simulink model "NREL_Diesel_Genset_Test_System"  (Simulink 8.1)
settings: Solver=ode3  SolverMode=SingleTasking  StartTime=0.0  StopTime=Stim.Trep  FixedStep=Ts  RelTol=1e-3
PostLoadFcn:
  | Ts=100e-6;GenSelect='3.5MW';initGTS;
InitFcn:
  | Ts=100e-6;GenSelect='3.5MW';initGTS;
values from neighbouring files (symbols this model uses):
  GenMult = 1    [initGTS.m]
  GenPN = 3.5e6    (= 3500000)    [initGTS.m]
  GenVN = 13800    [initGTS.m]
undefined symbols (not defined in the file or in its folder): breakers_1ph_3ph, CBID, DER_REL, DiscIntNeverNeededParam, Efd0, Efd1, Efd2, F3, Gen_900kW_external_control, HIL_GenSet, Ka, Ke, Kf, Protection, SeEfd1, SeEfd2, Stim, Ta, Te, Tf, VR0, VRmax, VRmin
libraries: powerlib x33, powerlib_extras x10, simulink x9, PQFV_lib x2, rtlab x2, cables_lib x2, breaker_lib x2, NREL_Diesel_Genset_lib x2, relay_modbus_lib x2, powerlib_models x1
(part 2 of 2)

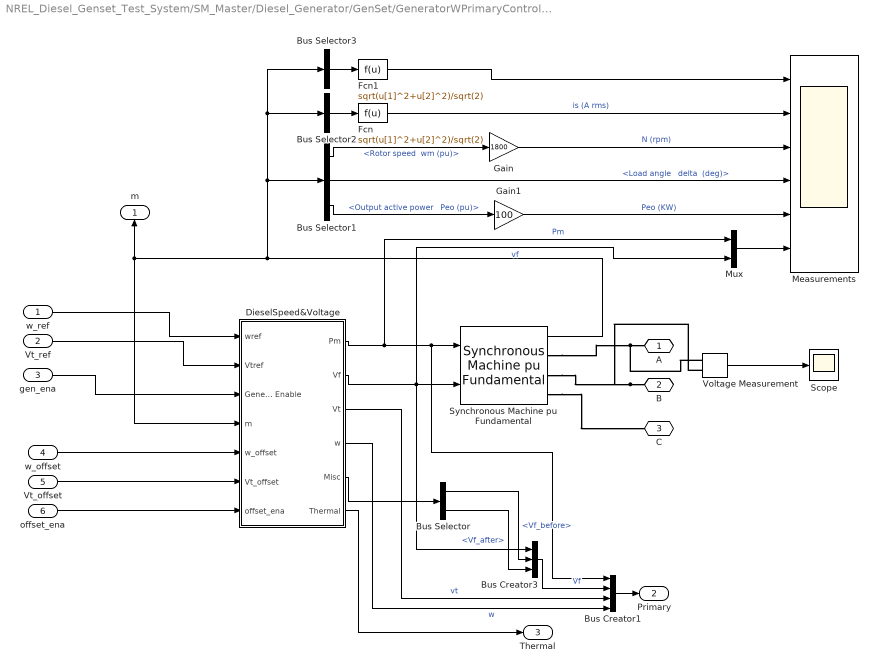
== system NREL_Diesel_Genset_Test_System/SM_Master/Diesel_Generator/GenSet/GeneratorWPrimaryControllers ==
  w_ref : Inport
  Vt_ref : Inport  Port=2
  gen_ena : Inport  Port=3
  w_offset : Inport  Port=4
  Vt_offset : Inport  Port=5
  offset_ena : Inport  Port=6
  Bus Creator1 : BusCreator
  Bus Creator3 : BusCreator  Inputs=3
  Bus Selector : BusSelector  OutputSignals=Vf_before,Vf_after
  Bus Selector1 : BusSelector  OutputSignals="Mechanical.Rotor speed  wm (pu),Load angle   delta  (deg),Output active power   Peo (pu)"
  Bus Selector2 : BusSelector  OutputSignals="dq0 components.Stator current  iq (pu),dq0 components.Stator current  id (pu)"  OutputAsBus=on
  Bus Selector3 : BusSelector  OutputSignals="dq0 components.Stator voltage  vq (pu),dq0 components.Stator voltage  vd (pu)"  OutputAsBus=on
  DieselSpeed&Voltage : Subsystem
  Fcn : Fcn  Expr=sqrt(u[1]^2+u[2]^2)/sqrt(2)
  Fcn1 : Fcn  Expr=sqrt(u[1]^2+u[2]^2)/sqrt(2)
  Gain : Gain  Gain=1800  SaturateOnIntegerOverflow=on  OutDataTypeStr=Inherit: Same as input  ParamDataTypeStr=Inherit: Same as input
  Gain1 : Gain  Gain=100  SaturateOnIntegerOverflow=on  OutDataTypeStr=Inherit: Same as input  ParamDataTypeStr=Inherit: Same as input
  Measurements : Scope  NumInputPorts=6
      settings: TickLabels=on  TimeRange=3  YMin=0~0~0~-200~-2.5e+18~-0.05  YMax=7e+08~1e+08~2.75e+08~200~1.25e+19~0.2  SaveName=is
  Mux : Mux  Inputs=2
  Scope : Scope
      settings: YMin=-750  YMax=750  SaveName=ScopeData12  Decimation=10
  Synchronous Machine pu Fundamental : powerlib/Machines/Synchronous Machine pu Fundamental  PresetModel=No  MechanicalLoad=Mechanical power Pm  ShowDetailedParameters=on  RotorType=Salient-pole  NominalParameters=[GP.Pn GP.Vn GP.fn]  Stator=GP.Stator  Field=GP.Field  Dampers2=[0.0652, 0.5134, 0.0287, 0.2553, 7.765e-3, 0.9167 ]  Dampers1=GP.Dampers  Mechanical=GP.Inertia  PolePairs=2  InitialConditions=GP.Initial  SetSaturation=off  Saturation=[0.6404,0.7127,0.8441,0.9214,0.9956,1.082,1.19,1.316,1.457;0.7,0.7698,0.8872,0.9466,0.9969,1.046,1.1,1.151,1.201]  Units=per unit fundamental parameters  LoadFlowParameters=[1,0,0,0,0]  TsPowergui=0  TsBlock=-1  IterativeModel=Trapezoidal non iterative  BusType=swing  Pref=0  Qref=0  Qmin=-inf  Qmax=inf  PLF=0  QLF=0
  Voltage Measurement : powerlib/Measurements/Voltage Measurement  PhasorSimulation=off  OutputType=Complex  PSBequivalent=0
  A : PMIOPort  Port=1  Side=Right
  B : PMIOPort  Port=2  Side=Right
  C : PMIOPort  Port=3  Side=Right
  m : Outport
  Primary : Outport  Port=2
  Thermal : Outport  Port=3
  wires:
  offset_ena/1 -> DieselSpeed&Voltage/7(offset_ena)
  Vt_offset/1 -> DieselSpeed&Voltage/6(Vt_offset)
  w_offset/1 -> DieselSpeed&Voltage/5(w_offset)
  Voltage Measurement/1 -> Scope/1
  Mux/1 -> Measurements/6
  Fcn1/1 -> Measurements/1
  Bus Selector3/1 -> Fcn1/1
  Bus Selector1/1 -> Gain/1  "<Rotor speed  wm (pu)>"
  Bus Selector1/2 -> Measurements/4  "<Load angle   delta  (deg)>"
  Bus Selector1/3 -> Gain1/1  "<Output active power   Peo (pu)>"
  Gain1/1 -> Measurements/5  "Peo (KW)"
  Gain/1 -> Measurements/3  "N (rpm)"
  Bus Selector2/1 -> Fcn/1
  Fcn/1 -> Measurements/2  "is (A rms)"
  Vt_ref/1 -> DieselSpeed&Voltage/2(Vtref)
  w_ref/1 -> DieselSpeed&Voltage/1(wref)
  DieselSpeed&Voltage/2(Vf) -> Synchronous Machine pu Fundamental/2, Mux/2, Bus Creator3/1  "vf"
  DieselSpeed&Voltage/1(Pm) -> Bus Creator1/1, Synchronous Machine pu Fundamental/1, Mux/1  "Pm"
  gen_ena/1 -> DieselSpeed&Voltage/3(Generator Enable)
  Synchronous Machine pu Fundamental/1 -> m/1, DieselSpeed&Voltage/4(m), Bus Selector3/1, Bus Selector2/1, Bus Selector1/1
  DieselSpeed&Voltage/3(Vt) -> Bus Creator1/3  "vt"
  DieselSpeed&Voltage/4(w) -> Bus Creator1/4  "w"
  Bus Creator1/1 -> Primary/1
  DieselSpeed&Voltage/5(Misc) -> Bus Selector/1
  Bus Selector/1 -> Bus Creator3/2  "<Vf_before>"
  Bus Selector/2 -> Bus Creator3/3  "<Vf_after>"
  Bus Creator3/1 -> Bus Creator1/2  "Vf"
  DieselSpeed&Voltage/6(Thermal) -> Thermal/1
  connections:
  Synchronous Machine pu Fundamental/RConn3 -- C/RConn1
  B/RConn1 -- Voltage Measurement/LConn2 -- Synchronous Machine pu Fundamental/RConn2
  A/RConn1 -- Voltage Measurement/LConn1 -- Synchronous Machine pu Fundamental/RConn1

== system NREL_Diesel_Genset_Test_System/SM_Master/Diesel_Generator/GenSet/NumOscillation ==
  Ground2 : powerlib/Elements/Ground  LConnTagsString=a
  "RLC " : powerlib/Elements/Parallel RLC Branch  LConnTagsString=a  RConnTagsString=__new0  BranchType=R  Resistance=10e6  Inductance=inf  SetiL0=off  InitialCurrent=0  Capacitance=10e-6  Setx0=off  InitialVoltage=0  Measurements=None
  RLC1 : powerlib/Elements/Parallel RLC Branch  LConnTagsString=a  RConnTagsString=__new0  BranchType=R  Resistance=10e6  Inductance=inf  SetiL0=off  InitialCurrent=0  Capacitance=10e-6  Setx0=off  InitialVoltage=0  Measurements=None
  RLC2 : powerlib/Elements/Parallel RLC Branch  LConnTagsString=a  RConnTagsString=__new0  BranchType=R  Resistance=10e6  Inductance=inf  SetiL0=off  InitialCurrent=0  Capacitance=10e-6  Setx0=off  InitialVoltage=0  Measurements=None
  RLC3 : powerlib/Elements/Parallel RLC Branch  LConnTagsString=a  RConnTagsString=__new0  BranchType=R  Resistance=10e-3  Inductance=inf  SetiL0=off  InitialCurrent=0  Capacitance=0  Setx0=off  InitialVoltage=0  Measurements=None
  RLC4 : powerlib/Elements/Parallel RLC Branch  LConnTagsString=a  RConnTagsString=__new0  BranchType=R  Resistance=10e-3  Inductance=inf  SetiL0=off  InitialCurrent=0  Capacitance=0  Setx0=off  InitialVoltage=0  Measurements=None
  RLC5 : powerlib/Elements/Parallel RLC Branch  LConnTagsString=a  RConnTagsString=__new0  BranchType=R  Resistance=10e-3  Inductance=inf  SetiL0=off  InitialCurrent=0  Capacitance=0  Setx0=off  InitialVoltage=0  Measurements=None
  A : PMIOPort  Port=1  Side=Left
  B : PMIOPort  Port=2  Side=Left
  C : PMIOPort  Port=3  Side=Left
  connections:
  C/RConn1 -- RLC5/LConn1
  B/RConn1 -- RLC4/LConn1
  A/RConn1 -- RLC3/LConn1
  RLC3/RConn1 -- RLC2/LConn1
  RLC1/LConn1 -- RLC4/RConn1
  "RLC "/LConn1 -- RLC5/RConn1
  RLC2/RConn1 -- Ground2/LConn1 -- RLC1/RConn1 -- "RLC "/RConn1

== system NREL_Diesel_Genset_Test_System/SM_Master/Diesel_Generator/GenSet/StabilityL ==
  Constant Load : powerlib/Elements/Three-Phase Parallel RLC Load  LConnTagsString=A|B|C  Configuration=Y (grounded)  NominalVoltage=v  NominalFrequency=60  ActivePower=kVA*1E3*pf  InductivePower=kVA*1E3*sqrt(1-pf^2)  CapacitivePower=0  Measurements=None  LoadType=constant Z
  A : PMIOPort  Port=1  Side=Left
  B : PMIOPort  Port=2  Side=Left
  C : PMIOPort  Port=3  Side=Left
  connections:
  A/RConn1 -- Constant Load/LConn1
  B/RConn1 -- Constant Load/LConn2
  C/RConn1 -- Constant Load/LConn3

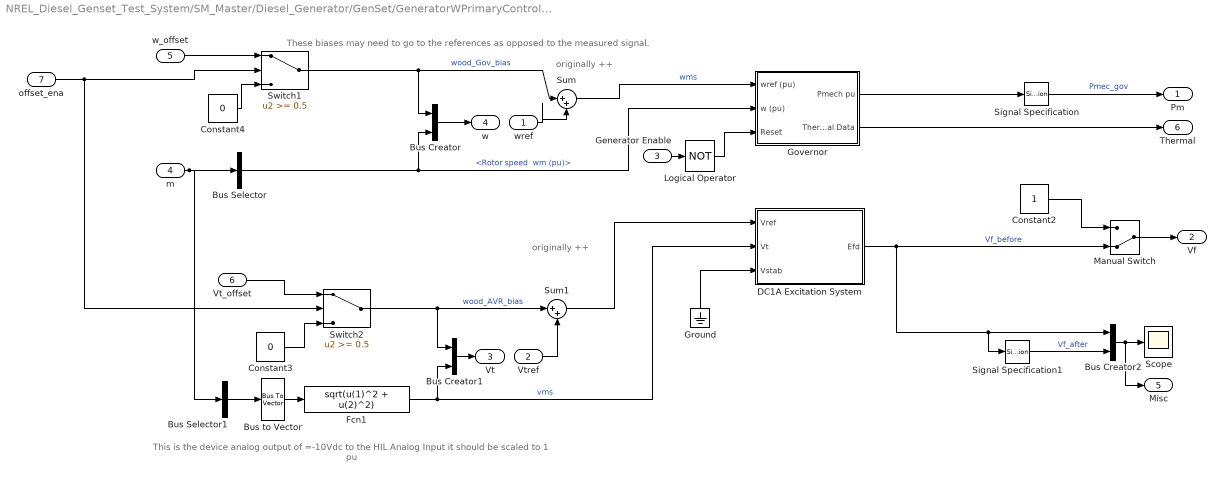
== system NREL_Diesel_Genset_Test_System/SM_Master/Diesel_Generator/GenSet/GeneratorWPrimaryControllers/DieselSpeed&Voltage ==
  note: This is the device analog output of =-10Vdc to
      | the HIL Analog Input it should be scaled to 1 pu
  note: These biases may need to
      | go to the references as opposed
      | to the measured signal.
  note: originally ++
  note: originally ++
  wref : Inport  SampleTime=Ts
  Vtref : Inport  Port=2  SampleTime=Ts
  Generator Enable : Inport  Port=3  SampleTime=Ts
  m : Inport  Port=4  SampleTime=Ts
  w_offset : Inport  Port=5
  Vt_offset : Inport  Port=6
  offset_ena : Inport  Port=7
  Bus Creator : BusCreator  Inputs=2
  Bus Creator1 : BusCreator  Inputs=2
  Bus Creator2 : BusCreator  Inputs=2
  Bus Selector : BusSelector  OutputSignals="Mechanical.Rotor speed  wm (pu)"
  Bus Selector1 : BusSelector  OutputSignals="dq0 components.Stator voltage  vd (pu),dq0 components.Stator voltage  vq (pu)"  OutputAsBus=on
  Bus to Vector : BusToVector
  Constant2 : Constant
  Constant3 : Constant  Value=0
  Constant4 : Constant  Value=0
  DC1A Excitation System : Subsystem  AncestorBlock=sps_avr/DC1A Excitation System  mask(DC1A Excitation System){Tr=GP.Ex.Tr, KaTa=GP.Ex.Regulator, VRminmax=[0 8], KfTf=GP.Ex.Damping, TbTc=[0 0], KeTe=GP.Ex.Exciter, Efd12=[6.83 6.08], SeEfd12=[ 0.132 0.062], v0=[0 0], TsBlock=Ts}
      mask prompts: Tr "Low-pass filter time constant Tr(s):"; KaTa "Voltage regulator gain and time constant [Ka Ta(s)]:"; VRminmax "Voltage regulator output limits [VRmin(pu) VRmax(pu)]:"; KfTf "Damping filter gain and time constant [Kf Tf(s)]:"; TbTc "Transient gain reduction lead and lag time constants [Tb(s) Tc(s)]:"; KeTe "Exciter gain and time constant [Ke Te(s)]:"; Efd12 "Field voltage values [Efd1(pu) Efd2(pu)]:"; SeEfd12 "Exciter saturation function values [SeEfd1(pu) SeEfd2(pu)]:"; v0 "Initial values of terminal voltage and field voltage [Vt0(pu) Efd0(pu)]:"; TsBlock "Sample time:"
      mask help: Implements a synchronous machine voltage regulator and exciter based on the IEEE type DC1A excitation system model. The output is the field voltage to apply to the Vf input of a Synchronous Machine block. Inputs and output are in p.u.
      mask init:
      | block = gcb;
      | [Ts,BlockChoice,MaskType,Ka,Ta,Ke,Te,Kf,Tf,Tb,Tc,Efd1,Efd2,SeEfd1,SeEfd2,VRmin,VRmax,Vt0,Efd0,VR0] = powericon('ExcitationSystemInit',block,TsBlock,KaTa,KeTe,KfTf,TbTc,Efd12,SeEfd12,VRminmax,v0);
      | %powericon('SetInternalModels','set',block,BlockChoice);
      mask Help: helpview(psbhelp);
      mask Display: color('blue');disp('DC1A')
  Fcn1 : Fcn  Expr=sqrt(u(1)^2 + u(2)^2)
  Governor : Subsystem  BlockChoice=GEJenbacherJ620
      settings: AttributesFormatString=%<BlockChoice>  MemberBlocks=DieselGovernor,GEJenbacherJ620
      settings: TemplateBlock=|
      | NREL_Diesel_Genset_lib/Configurable
      | Subsystem
  Ground : Ground
  Logical Operator : Logic  Operator=NOT  AllPortsSameDT=off  OutDataTypeStr=boolean
  Manual Switch : ManualSwitch  CurrentSetting=0
  Scope : Scope
      settings: YMin=1.0475  YMax=1.08
  Signal Specification : SignalSpecification  Dimensions=1
  Signal Specification1 : SignalSpecification  Dimensions=1
  Sum : Sum  Inputs=|++
  Sum1 : Sum  Inputs=|++
  Switch1 : Switch  Threshold=0.5
  Switch2 : Switch  Threshold=0.5
  Pm : Outport
  Vf : Outport  Port=2
  Vt : Outport  Port=3
  w : Outport  Port=4
  Misc : Outport  Port=5
  Thermal : Outport  Port=6
  wires:
  Constant3/1 -> Switch2/3
  Constant4/1 -> Switch1/3
  w_offset/1 -> Switch1/1
  offset_ena/1 -> Switch2/2, Switch1/2
  Vt_offset/1 -> Switch2/1
  Manual Switch/1 -> Vf/1
  Constant2/1 -> Manual Switch/1
  Generator Enable/1 -> Logical Operator/1
  Bus to Vector/1 -> Fcn1/1
  Bus Selector1/1 -> Bus to Vector/1
  m/1 -> Bus Selector1/1, Bus Selector/1
  Bus Selector/1 -> Bus Creator/2, Governor/2(w (pu))  "<Rotor speed  wm (pu)>"
  Fcn1/1 -> DC1A Excitation System/2(Vt), Bus Creator1/2  "vms"
  Ground/1 -> DC1A Excitation System/3(Vstab)
  Bus Creator/1 -> w/1
  Bus Creator1/1 -> Vt/1
  DC1A Excitation System/1(Efd) -> Signal Specification1/1, Bus Creator2/1, Manual Switch/2  "Vf_before"
  Bus Creator2/1 -> Scope/1, Misc/1
  Switch1/1 -> Sum/1, Bus Creator/1  "wood_Gov_bias"
  Switch2/1 -> Sum1/1, Bus Creator1/1  "wood_AVR_bias"
  Vtref/1 -> Sum1/2
  Sum1/1 -> DC1A Excitation System/1(Vref)
  wref/1 -> Sum/2
  Sum/1 -> Governor/1(wref (pu))  "wms"
  Signal Specification/1 -> Pm/1  "Pmec_gov"
  Signal Specification1/1 -> Bus Creator2/2  "Vf_after"
  Logical Operator/1 -> Governor/3(Reset)
  Governor/1(Pmech pu) -> Signal Specification/1
  Governor/2(Thermal Data) -> Thermal/1

== system NREL_Diesel_Genset_Test_System/SM_Master/Diesel_Generator/GenSet/GeneratorWPrimaryControllers/DieselSpeed&Voltage/DC1A Excitation System ==
  Vref : Inport
  Vt : Inport  Port=2
  Vstab : Inport  Port=3
  Discrete : Subsystem  mask(Excitation System){}
  Efd : Outport
  wires:
  Vstab/1 -> Discrete/3(Vstab)
  Discrete/1(Efd) -> Efd/1
  Vt/1 -> Discrete/2(Vt)
  Vref/1 -> Discrete/1(Vref)

== system NREL_Diesel_Genset_Test_System/SM_Master/Diesel_Generator/GenSet/GeneratorWPrimaryControllers/DieselSpeed&Voltage/Governor ==
  wref (pu) : Inport
  w (pu) : Inport  Port=2
  Reset : Inport  Port=3
  GEJenbacherJ620 : NREL_Diesel_Genset_lib/GEJenbacherJ620  cd=.8  H=47133  keq=1.3962  Ma=.029  Meq=.0285  Mf=.019  P0=800000  Pm=37241  R=8.314  T0=300  Tm=325  thermalEfficiency=.45  V=0.031  Vd=0.125  volumeEfficiency=.9  P=3  I=3  UL=1.05  LL=0  UPL=1.5  LPL=0
  Pmech pu : Outport
  Thermal Data : Outport  Port=2
  wires:
  wref (pu)/1 -> GEJenbacherJ620/1
  w (pu)/1 -> GEJenbacherJ620/2
  Reset/1 -> GEJenbacherJ620/3
  GEJenbacherJ620/1 -> Pmech pu/1
  GEJenbacherJ620/2 -> Thermal Data/1

== system NREL_Diesel_Genset_Test_System/SM_Master/Diesel_Generator/GenSet/GeneratorWPrimaryControllers/DieselSpeed&Voltage/DC1A Excitation System/Discrete ==
  note: Vt0
  note: VR0/Ka
  note: VR0/Ka
  note: VR0/Ka
  note: VR0=Efd0*Se+Ke*Efd0
  note: Efd0
  note: Vt0
  note: Vt0
  note: Ke*Efd0
  note: Efd0
  note: Main Regulator
      | Ka/(Ta.s+1)
  note: Initial values are shown in blue
  note: 0
  note: VRmax
  note: VRmin
  note: __
      |              /
      |           /
      |         /
      |       /
      | __/
  note: Efd0*Se
  Vref : Inport
  Vt : Inport  Port=2
  Vstab : Inport  Port=3
  1/Te : Gain  Gain=1/Te
  Damping Filter Kf.s/(Tf.s+1) : Subsystem  mask{Kf=Kf, Tf=Tf, X0=Efd0*Kf/Tf}
      mask prompts: Kf "Damping filter gain Kf:"; Tf "Damping filter time constant Tf(s):"; X0 "Initial conditions:"
      mask Display: disp('Kfs\n---\n1+Tfs')
  Discrete PID Controller : simulink/Continuous/PID Controller  Controller=PID  TimeDomain=Discrete-time  SampleTime=Ts  IntegratorMethod=Forward Euler  FilterMethod=Forward Euler  Form=Parallel  P=1  I=1  D=0  N=100  InitialConditionSource=internal  InitialConditionForIntegrator=0  InitialConditionForFilter=0  ExternalReset=none  LimitOutput=on  UpperSaturationLimit=VRmax  LowerSaturationLimit=VRmin  LinearizeAsGain=off  AntiWindupMode=none  Kb=1  TrackingMode=off  Kt=1  PParamMin=[]  PParamMax=[]  IParamMin=[]  IParamMax=[]  DParamMin=[]  DParamMax=[]  NParamMin=[]  NParamMax=[]  KbParamMin=[]  KbParamMax=[]  KtParamMin=[]  KtParamMax=[]  POutMin=[]  POutMax=[]  IOutMin=[]  IOutMax=[]  DOutMin=[]  DOutMax=[]  NOutMin=[]  NOutMax=[]  KbOutMin=[]  KbOutMax=[]  KtOutMin=[]  KtOutMax=[]  IntegratorOutMin=[]  IntegratorOutMax=[]  FilterOutMin=[]  FilterOutMax=[]  SumOutMin=[]  SumOutMax=[]  SumI1OutMin=[]  SumI1OutMax=[]  SumI2OutMin=[]  SumI2OutMax=[]  SumI3OutMin=[]  SumI3OutMax=[]  SumDOutMin=[]  SumDOutMax=[]  SaturationOutMin=[]  SaturationOutMax=[]  IntegratorContinuousStateAttributes=''  IntegratorStateMustResolveToSignalObject=off  IntegratorRTWStateStorageClass=Auto  FilterContinuousStateAttributes=''  FilterStateMustResolveToSignalObject=off  FilterRTWStateStorageClass=Auto
  Discrete-Time Integrator : DiscreteIntegrator  InitialCondition=Efd0  SampleTime=Ts  LimitOutput=on  ICPrevOutput=DiscIntNeverNeededParam  ICPrevScaledInput=DiscIntNeverNeededParam
  Gain3 : Gain  Gain=Ke  SaturateOnIntegerOverflow=on  OutDataTypeStr=Inherit: Same as input  ParamDataTypeStr=Inherit: Same as input
  Low Pass Filter 1/(Tr.s+1) : powerlib_models/Discrete/Excitation_System/Low Pass Filter 1 // (tr.s +1) (with IC)  FilterType=Lowpass  Tc=Tr  Ts=Ts  Initialize=on  Vac_Init=[0 0 60]  Vdc_Init=Vt0  PlotResponse=off  param1=[1 500 0.1]
  Saturation Vx=Efd*Se[Efd] : Subsystem  mask{Efd12=[Efd1 Efd2], SeEfd12=[SeEfd1 SeEfd2]}
      mask prompts: Efd12 "Field voltage values [Efd1(pu) Efd2(pu)]:"; SeEfd12 "Exciter saturation function values [SeEfd1(pu) SeEfd2(pu)]:"
      mask init:
      | Efd1 = Efd12(1);Efd2 = Efd12(2);
      | SeEfd1 = SeEfd12(1);SeEfd2 = SeEfd12(2);
  Sum : Sum  Inputs=++-+-  SaturateOnIntegerOverflow=on  InputSameDT=on  OutDataTypeStr=Inherit: Same as first input
  Sum1 : Sum  Inputs=|+-
  Sum2 : Sum  Inputs=|++
  Transient Gain Reduction (Tc.s+1)/(Tb.s+1) : powerlib_extras/Discrete  Control Blocks/Discrete Lead-Lag  T1=Tc  T2=Tb  V_Init=VR0/Ka  Ts=Ts
  VR0/Ka : Constant  Value=VR0/Ka
  Vaminmax : Subsystem  mask{Ka=Ka, Ta=Ta, VRminmax=[VRmin VRmax], X0=VR0}
      mask prompts: Ka "Voltage regulator gain Ka:"; Ta "Voltage regulator time constant Ta(s):"; VRminmax "Voltage regulator output limits [VRmin(pu) VRmax(pu)]:"; X0 "Initial conditions:"
      mask init:
      | VRmin=VRminmax(1);VRmax=VRminmax(2);
      mask Display: disp('Ka\n---\n1+Tas')
  Efd : Outport
  wires:
  Vt/1 -> Low Pass Filter 1/(Tr.s+1)/1  "Vt"
  Gain3/1 -> Sum2/2
  Vstab/1 -> Sum/4
  Low Pass Filter 1/(Tr.s+1)/1 -> Sum/3  "Vt"
  VR0/Ka/1 -> Sum/2
  Vref/1 -> Sum/1
  1/Te/1 -> Discrete-Time Integrator/1
  Discrete-Time Integrator/1 -> Efd/1, Saturation Vx=Efd*Se[Efd]/1(Efd), Damping Filter Kf.s/(Tf.s+1)/1(u), Gain3/1  "Efd"
  Sum1/1 -> 1/Te/1  "Vf"
  Sum2/1 -> Sum1/2  "Vfe"
  Transient Gain Reduction (Tc.s+1)/(Tb.s+1)/1 -> Vaminmax/1(u), Discrete PID Controller/1
  Sum/1 -> Transient Gain Reduction (Tc.s+1)/(Tb.s+1)/1
  Vaminmax/1(y) -> Sum1/1  "VR"
  Saturation Vx=Efd*Se[Efd]/1(Vx) -> Sum2/1  "Vx"
  Damping Filter Kf.s/(Tf.s+1)/1(y) -> Sum/5  "Vf"

== system NREL_Diesel_Genset_Test_System/SM_Master/Diesel_Generator/GenSet/GeneratorWPrimaryControllers/DieselSpeed&Voltage/DC1A Excitation System/Discrete/Damping Filter Kf.s/(Tf.s+1) ==
  note: 0
  note: Efd0*Kf/Tf
  note: Efd0
  u : Inport
  Discrete 1st-Order Filter : powerlib_extras/Discrete  Control Blocks/Discrete 1st-Order Filter  FilterType=Highpass  Tc=Tf  Ts=Ts  Initialize=on  Vac_Init=[0 0 60]  Vdc_Init=Efd0*Kf/Tf  PlotResponse=off  param1=[1 500 0.1]
  Gain2 : Gain  Gain=Kf/Tf  SaturateOnIntegerOverflow=on  OutDataTypeStr=Inherit: Same as input  ParamDataTypeStr=Inherit: Same as input
  y : Outport
  wires:
  Gain2/1 -> Discrete 1st-Order Filter/1
  Discrete 1st-Order Filter/1 -> y/1
  u/1 -> Gain2/1

== system NREL_Diesel_Genset_Test_System/SM_Master/Diesel_Generator/GenSet/GeneratorWPrimaryControllers/DieselSpeed&Voltage/DC1A Excitation System/Discrete/Saturation Vx=Efd*Se[Efd] ==
  Efd : Inport
  Lookup Table : Lookup  InputValues=[0 Efd2 Efd1]  Table=[0 SeEfd2 SeEfd1]
  Product : Product  RndMeth=Zero
  Vx : Outport
  wires:
  Lookup Table/1 -> Product/2
  Product/1 -> Vx/1
  Efd/1 -> Lookup Table/1, Product/1

== system NREL_Diesel_Genset_Test_System/SM_Master/Diesel_Generator/GenSet/GeneratorWPrimaryControllers/DieselSpeed&Voltage/DC1A Excitation System/Discrete/Vaminmax ==
  note: VR0/Ka
  note: VR0
  note: VR0
  note: 0
  note: VR0
  u : Inport
  Discrete-Time Integrator : DiscreteIntegrator  InitialCondition=VR0  SampleTime=Ts  LimitOutput=on  UpperSaturationLimit=VRmax  LowerSaturationLimit=VRmin  ICPrevOutput=DiscIntNeverNeededParam  ICPrevScaledInput=DiscIntNeverNeededParam
  Gain1 : Gain  Gain=1/Ta  SaturateOnIntegerOverflow=on  OutDataTypeStr=Inherit: Same as input  ParamDataTypeStr=Inherit: Same as input
  Gain2 : Gain  Gain=Ka  SaturateOnIntegerOverflow=on  OutDataTypeStr=Inherit: Same as input  ParamDataTypeStr=Inherit: Same as input
  Sum : Sum  Inputs=|+-  SaturateOnIntegerOverflow=on  InputSameDT=on  OutDataTypeStr=Inherit: Same as first input
  y : Outport
  wires:
  u/1 -> Gain2/1
  Sum/1 -> Gain1/1
  Discrete-Time Integrator/1 -> y/1, Sum/2
  Gain2/1 -> Sum/1
  Gain1/1 -> Discrete-Time Integrator/1
